simulink model "Backsteping2_Tanques_2_Back"  (R2025b)
settings: Solver=VariableStepAuto  StartTime=0.0  StopTime=100  RelTol=1e-3
settings Model: Creator=HP  LastModifiedBy=ACER
settings SolverCC: AlgebraicLoopSolver=TrustRegion
settings DebuggingCC: UnconnectedInputMsg=warning  UnconnectedOutputMsg=warning  UnconnectedLineMsg=warning
settings ModelReferenceCC: EnableRefExpFcnMdlSchedulingChecks=on
settings RTWCC: GPUComputeCapability=3.5

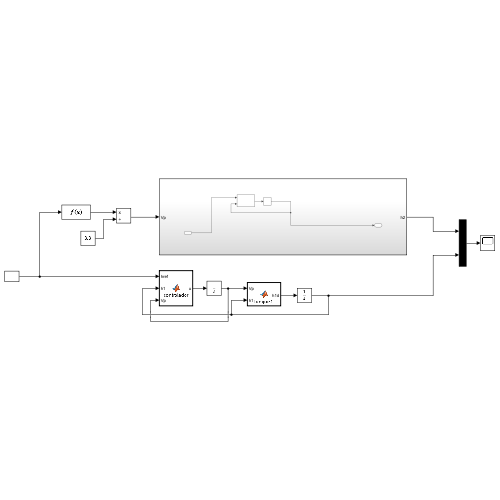
[thumbnail: Simulink's stored preview of the top-level diagram]
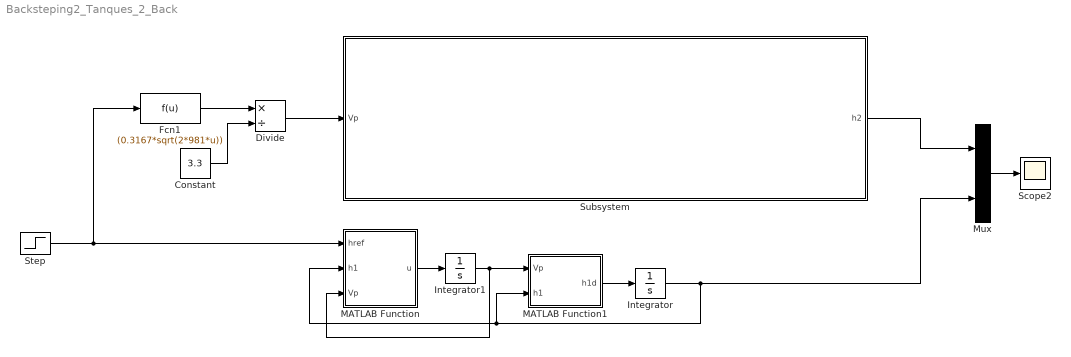
== system Backsteping2_Tanques_2_Back ==
  Constant : Constant  Value=3.3
  Divide : Product  Inputs=*/
  Fcn1 : Fcn  Expr=(0.3167*sqrt(2*981*u))
  Integrator : Integrator
  Integrator1 : Integrator
  MATLAB Function : MATLAB Function  TreatAsAtomicUnit=on
  MATLAB Function1 : MATLAB Function  TreatAsAtomicUnit=on
  Mux : Mux  Inputs=2
  Scope2 : Scope
      settings: ActiveDisplayYMinimum=-2.9999999999999991  ActiveDisplayYMaximum=27  DataLoggingVariableName=ScopeData2
  Step : Step  Time=0  After=10  SampleTime=0
  Subsystem : Subsystem
  wires:
  MATLAB Function1/1(h1d) -> Integrator/1
  Integrator/1 -> Mux/2, MATLAB Function/2(h1), MATLAB Function1/2(h1)
  Mux/1 -> Scope2/1
  MATLAB Function/1(u) -> Integrator1/1
  Integrator1/1 -> MATLAB Function/3(Vp), MATLAB Function1/1(Vp)
  Constant/1 -> Divide/2
  Divide/1 -> Subsystem/1(Vp)
  Fcn1/1 -> Divide/1
  Step/1 -> MATLAB Function/1(href), Fcn1/1
  Subsystem/1(h2) -> Mux/1

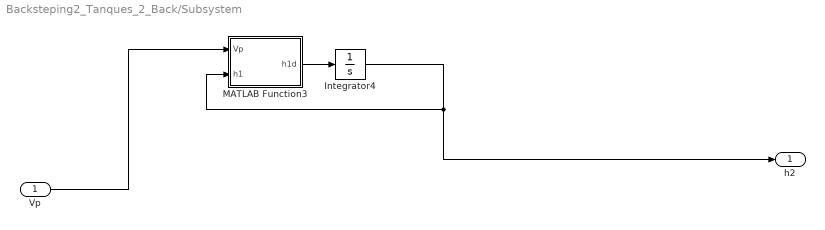
== system Backsteping2_Tanques_2_Back/Subsystem ==
  Vp : Inport
  Integrator4 : Integrator
  MATLAB Function3 : MATLAB Function  TreatAsAtomicUnit=on
  h2 : Outport
  wires:
  MATLAB Function3/1(h1d) -> Integrator4/1
  Vp/1 -> MATLAB Function3/1(Vp)
  Integrator4/1 -> h2/1, MATLAB Function3/2(h1)

== matlab function Backsteping2_Tanques_2_Back/MATLAB Function1 ==
  data: Vp input; h1d output; h1 input
function h1d = tanque1(Vp, h1)
% Parametros
dt1=4.445; %cm
d01=0.635; %cm
At1=pi*dt1^2/4;  % ajustar
A01=pi*d01^2/4;
Kp=3.3;            %cm3/(s*V)
g=980;  % cm/s2

A = Kp/At1;
B = sqrt(2*g)*A01/At1;

h1_fr = abs(h1);

% modelo no lineal A*dL1/dt=Fi1 - F01
h1d=A*Vp-B*sqrt(h1_fr);

== matlab function Backsteping2_Tanques_2_Back/MATLAB Function ==
  data: href input; h1 input; u output; Vp input
function u = controlador(href, h1, Vp)
% Backstepping 1 tanque (u = dVp/dt) con TUS PARÁMETROS
% Entradas:
%   href : altura deseada (cm)
%   h1   : altura medida (cm)
%   Vp   : voltaje actual de la bomba (V)
%
% Salida:
%   u    : dVp/dt (V/s)  --> va al integrador 1/s para obtener Vp

% ----- TUS DATOS (cm, s, V) -----
dt1 = 4.445;                 % diámetro tanque [cm]
d01 = 0.635;                 % diámetro orificio [cm]
At1 = pi*dt1^2/4;            % A1 (área del tanque)
A01 = pi*d01^2/4;            % Ao1 (área del orificio)
g   = 980;                   % gravedad [cm/s^2]
Kp  = 3.3;                   % ganancia de la bomba
k   = 1.0;                   % GANANCIA de paso 3 (ajústala >0)

% ----- Protecciones numéricas -----
epsh = 1e-3;                 % evita sqrt(0) y divisiones
x  = max(abs(h1), epsh);     % x = h1 >= eps
r  = max(href, 0);           % referencia no negativa
e  = x - r;                  % error
xi = Vp;                     % xi = Vp (feedback del integrador de Vp)

% ----- Dinámica del tanque: xdot = f(x) + g(x)*xi -----
fx = -(A01/At1) * sqrt(2*g*x);
gx =  (Kp/At1);

% ----- Control virtual (tracking): phi(e,r) y su derivada -----
% Nota: como e+r = x, usamos x directamente en la raíz para mayor robustez
phi    = (A01/Kp)*sqrt(2*g*x) - (At1/Kp)*e;
dphide = (A01*sqrt(2*g))/(2*Kp*sqrt(x)) - (At1/Kp);

% ----- TU LEY DE CONTROL (de la diapositiva) -----
% u = (∂phi/∂e)*[ f(x)+g(x)*xi ] - [ e*g(x) + k*(xi - phi) ]
u = dphide*(fx + gx*xi) - ( e*gx + k*(xi - phi) );

% Seguridad numérica
if ~isfinite(u)
    u = 0;
end

== matlab function Backsteping2_Tanques_2_Back/Subsystem/MATLAB Function3 ==
  data: Vp input; h1d output; h1 input
function h1d = tanque1(Vp, h1)
% Parametros
dt1=4.445; %cm
d01=0.635; %cm
At1=pi*dt1^2/4;  % ajustar
A01=pi*d01^2/4;
Kp=3.3;   %cm3/(s*V)
g=980;  % cm/s2

A = Kp/At1;
B = sqrt(2*g)*A01/At1;

h1_fr = abs(h1);

% modelo no lineal A*dL1/dt=Fi1 - F01
h1d=A*Vp-B*sqrt(h1_fr);
